simulink model "Nonlinear_System"  (R2022b)
settings: Solver=daessc  StartTime=0.0  StopTime=9.9999375  MaxStep=1e-4  RelTol=1e-3  AbsTol=1e-3
InitFcn:
  | load('vars')
values from neighbouring files (symbols this model uses):
  Re = 7.62    [vars.mat]
libraries: nesl_utility x6, acoustical_lib x4, fl_lib x3, SpeakerSubsystemLibrary_1_0_0 x1
settings Model: Creator=sct12  LastModifiedBy=yuvalkonforti
settings SolverCC: AutoScaleAbsTol=off  AlgebraicLoopSolver=TrustRegion  MaxZcPerStep=1
settings DebuggingCC: UnconnectedInputMsg=warning  UnconnectedOutputMsg=warning  UnconnectedLineMsg=warning  SymbolicDimsDataTypeCodeGenerationDiagnostic=none  SFMachineParentedDataDiag=warning
settings ModelReferenceCC: EnableRefExpFcnMdlSchedulingChecks=on
settings SFSimCC: CustomCodeUndefinedFunction=UseInterfaceOnly
settings RTWCC: DLArmComputeVersion=19.05
settings SimscapeCC: SimscapeLogType=all  SimscapeLogSimulationStatistics=on  SimscapeLogDataHistory=10000

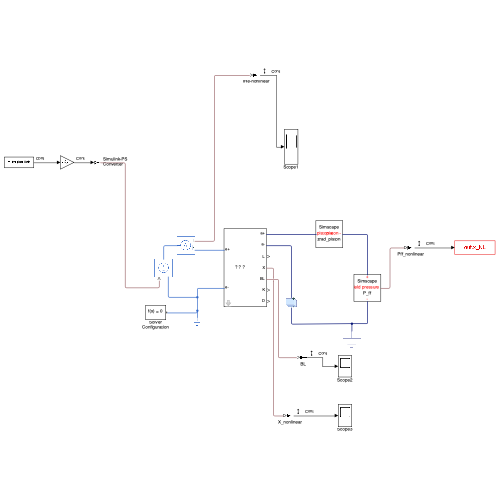
[thumbnail: Simulink's stored preview of the top-level diagram]
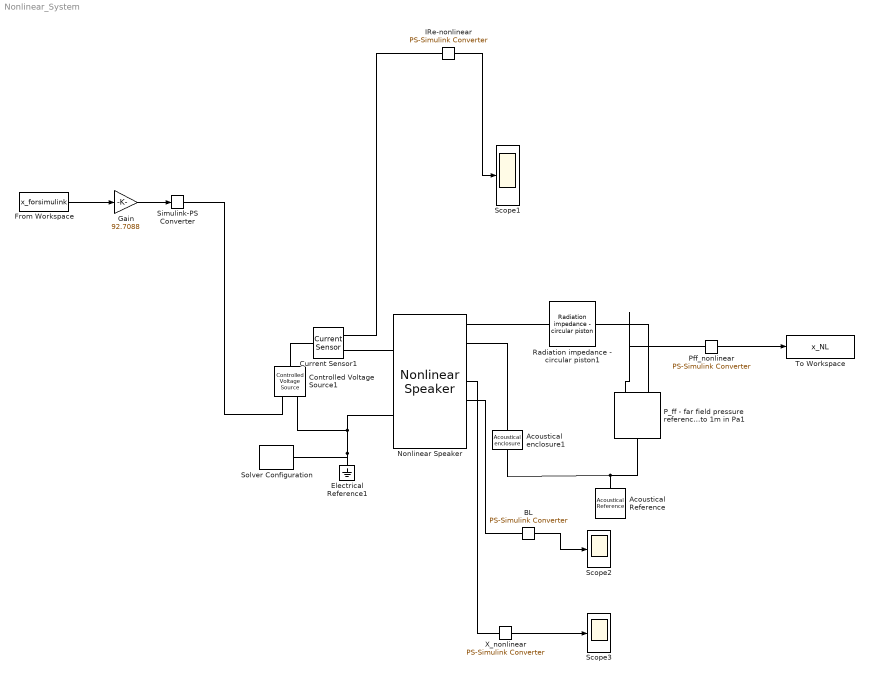
== system Nonlinear_System ==
  Acoustical Reference : acoustical_lib/Acoustical Elements/Acoustical Reference
      settings: InternalSimscapePortConfiguration="{\"Bottom\":[],\"Left\":[{\"id\":\"pp\",\"label\":\"\",\"type\":\"acoustical.acoustical\"}],\"Right\":[],\"Top\":[]}"
  Acoustical enclosure1 : acoustical_lib/Acoustical Elements/Acoustical enclosure  vol=1.5 l  u_specify=off  u_priority=None  u=0 m^3/s  u_nominal_specify=off  u_nominal_unit=m^3/s  u_nominal_value=1  p_specify=off  p_priority=None  p=0 Pa  p_nominal_specify=off  p_nominal_unit=Pa  p_nominal_value=1
      settings: InternalSimscapePortConfiguration="{\"Bottom\":[],\"Left\":[{\"id\":\"pp\",\"label\":\"+\",\"type\":\"acoustical.acoustical\"}],\"Right\":[{\"id\":\"nn\",\"label\":\"-\",\"type\":\"acoustical.acoustical\"}],\"Top\":[]}"
  BL : nesl_utility/PS-Simulink Converter  PhysicalDomain=network_engine_domain  SubClassName=ps_output  LeftPortType=input  RightPortType=output  PseudoPeriodic=off  Frequencies=[]  VectorFormat=inherit  Unit=inherit  AffineConversion=off
  Controlled Voltage Source1 : fl_lib/Electrical/Electrical Sources/Controlled Voltage Source
  Current Sensor1 : fl_lib/Electrical/Electrical Sensors/Current Sensor
  Electrical Reference1 : fl_lib/Electrical/Electrical Elements/Electrical Reference
  From Workspace : FromWorkspace  VariableName=x_forsimulink  SampleTime=-1
  Gain : Gain  Gain=92.7088
  IRe-nonlinear : nesl_utility/PS-Simulink Converter  PhysicalDomain=network_engine_domain  SubClassName=ps_output  LeftPortType=input  RightPortType=output  PseudoPeriodic=off  Frequencies=[]  VectorFormat=inherit  Unit=inherit  AffineConversion=off
  Nonlinear Speaker : SpeakerSubsystemLibrary_1_0_0/Nonlinear Speaker  Sd=Sd m^2  mass=Mm kg  R=Re Ohm  L2=L2 H  R2=R2 Ohm  L0_of_x=Le_0 H  L1_of_x=Le_1 H/m  L2_of_x=Le_2 H/m^2  L3_of_x=Le_3 H/m^3  L4_of_x=Le_4 H/m^4  Bl0=BL_0 N/A  Bl1=BL_1 N/(A*m)  Bl2=BL_2 N/(A*m^2)  Bl3=BL_3 N/(A*m^3)  Bl4=BL_4 N/(A*m^4)  K0=K_0 N/m  K1=K_1 N/m^2  K2=K_2 N/m^3  K3=K_3 N/m^4  K4=K_4 N/m^5  D0=D_0 N*s/m  D1=D_1 N*s^2/m^2  D2=D_2 N*s^3/m^3  D3=D_3 N*s^4/m^4  D4=D_4 N*s^5/m^5
  P_ff - far field pressure referenced to 1m in Pa1 : acoustical_lib/Acoustical Elements/P_ff - far field pressure referenced to 1m in Pa  dist=6.0323 m  u_specify=off  u_priority=None  u=0 m^3/s  u_nominal_specify=off  u_nominal_unit=m^3/s  u_nominal_value=1  p_specify=off  p_priority=None  p=0 Pa  p_nominal_specify=off  p_nominal_unit=Pa  p_nominal_value=1
      settings: InternalSimscapePortConfiguration="{\"Bottom\":[],\"Left\":[{\"id\":\"pp\",\"label\":\"+\",\"type\":\"acoustical.acoustical\"}],\"Right\":[{\"id\":\"nn\",\"label\":\"-\",\"type\":\"acoustical.acoustical\"}],\"Top\":[{\"id\":\"p_ff\",\"label\":\"far field pressure\",\"type\":\"output\"}]}"
  Pff_nonlinear : nesl_utility/PS-Simulink Converter  PhysicalDomain=network_engine_domain  SubClassName=ps_output  LeftPortType=input  RightPortType=output  PseudoPeriodic=off  Frequencies=[]  VectorFormat=inherit  Unit=inherit  AffineConversion=off
  Radiation impedance - circular piston1 : acoustical_lib/Acoustical Elements/Radiation impedance - circular piston  Sd=Sd m^2
      settings: InternalSimscapePortConfiguration="{\"Bottom\":[],\"Left\":[{\"id\":\"pa\",\"label\":\"piston +\",\"type\":\"acoustical.acoustical\"}],\"Right\":[{\"id\":\"na\",\"label\":\"piston -\",\"type\":\"acoustical.acoustical\"}],\"Top\":[]}"
  Scope1 : Scope
  Scope2 : Scope
  Scope3 : Scope
  Simulink-PS Converter : nesl_utility/Simulink-PS Converter  PhysicalDomain=network_engine_domain  SubClassName=ps_input  LeftPortType=input  RightPortType=output  PseudoPeriodic=off  Frequencies=[]  NoiseDistribution=none  NoiseParameters=[]  Unit=1  AffineConversion=off  FilteringAndDerivatives=filter  SimscapeFilterOrder=1  InputFilterTimeConstant=0.000001  UdotUserProvided=0
  Solver Configuration : nesl_utility/Solver Configuration  PhysicalDomain=network_engine_domain  SubClassName=solver  LeftPortType=input  RightPortType=generic  Tones=[]  Harmonics=[]  SimulateNoise=off  Profile=off  UseLocalSampling=off  EnableSwitchedLinearOptims=on  FrequencyDomain=off  UseCCode=off  RelTol=0.001  AbsTol=1e-06  MinStep=1e-09  ToWorkspace=off  RevertToSquareIcSolve=off  NumHomotopyIterations=100  PhasorMode=off  PhasorModeNumHarmonics=1  ConsistencySolver=NEWTON_XTOL_AFTER_FTOL  IndexReductionMethod=DerivativeReplacement  DoDC=off  ResidualTolerance=1e-09  ConsistencyTolSource=GLOBAL  ConsistencyAbsTol=0.001  ConsistencyRelTol=0.001  ConsistencyTolFactor=0.001  UseLocalSolver=off  LocalSolverChoice=NE_BACKWARD_EULER_ADVANCER  ResolveIndetEquations=on  FunctionEvalNumThread=1  LocalSolverSampleTime=0.001  DoFixedCost=off  MaxNonlinIter=3  MaxModeIter=2  ComputeImpulses=off  ImpulseIterations=2  LinearAlgebra=auto  LinearAlgebraNumThread=0  EquationFormulation=NE_TIME_EF  DelaysMemoryBudget=1024  AutomaticFiltering=on  FilteringTimeConstant=0.001  PartitionStorageMethod=AS_NEEDED  PartitionMemoryBudget=1024  PartitionMethod=ROBUST
  To Workspace : ToWorkspace  VariableName=x_NL  SampleTime=0.0000625
  X_nonlinear : nesl_utility/PS-Simulink Converter  PhysicalDomain=network_engine_domain  SubClassName=ps_output  LeftPortType=input  RightPortType=output  PseudoPeriodic=off  Frequencies=[]  VectorFormat=inherit  Unit=inherit  AffineConversion=off
  wires:
  Pff_nonlinear/1 -> To Workspace/1
  From Workspace/1 -> Gain/1
  IRe-nonlinear/1 -> Scope1/1
  Gain/1 -> Simulink-PS Converter/1
  BL/1 -> Scope2/1
  X_nonlinear/1 -> Scope3/1
  connections:
  P_ff - far field pressure referenced to 1m in Pa1/LConn1 -- Radiation impedance - circular piston1/RConn1
  Acoustical Reference/LConn1 -- P_ff - far field pressure referenced to 1m in Pa1/RConn1 -- Acoustical enclosure1/RConn1
  Radiation impedance - circular piston1/LConn1 -- Nonlinear Speaker/RConn1
  Nonlinear Speaker/LConn1 -- Current Sensor1/RConn2
  Controlled Voltage Source1/LConn1 -- Current Sensor1/LConn1
  Controlled Voltage Source1/RConn2 -- Nonlinear Speaker/LConn2 -- Solver Configuration/RConn1 -- Electrical Reference1/LConn1
  Controlled Voltage Source1/RConn1 -- Simulink-PS Converter/RConn1
  P_ff - far field pressure referenced to 1m in Pa1/LConn2 -- Pff_nonlinear/LConn1
  IRe-nonlinear/LConn1 -- Current Sensor1/RConn1
  Acoustical enclosure1/LConn1 -- Nonlinear Speaker/RConn2
  BL/LConn1 -- Nonlinear Speaker/RConn5
  Nonlinear Speaker/RConn4 -- X_nonlinear/LConn1
